simulink model "model1"  (R2023a)
settings: Solver=VariableStepAuto  StartTime=0.0  StopTime=2  RelTol=1e-5
values from neighbouring files (symbols this model uses):
  beta = 0.001    [LR1.m]
  C_m = 1.3    [LR1.m]
  C_w = 3.15    [LR1.m]
  J = 7e-6    (= 7e-06)    [LR1.m]
  L_ov = 0.013    [LR1.m]
  L_ya = 0.0015    [LR1.m]
  R_ya = 8    [LR1.m]
settings Model: Creator=Артём  LastModifiedBy=Артём

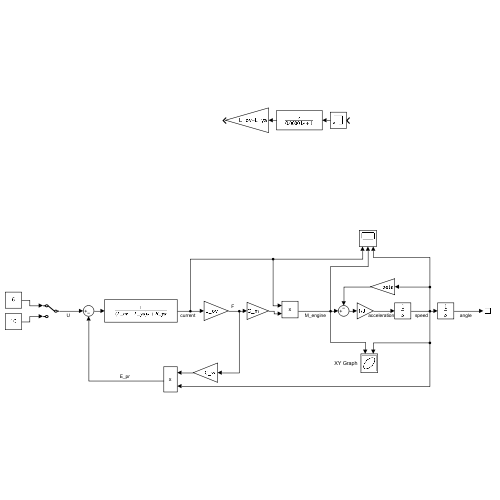
[thumbnail: Simulink's stored preview of the top-level diagram]
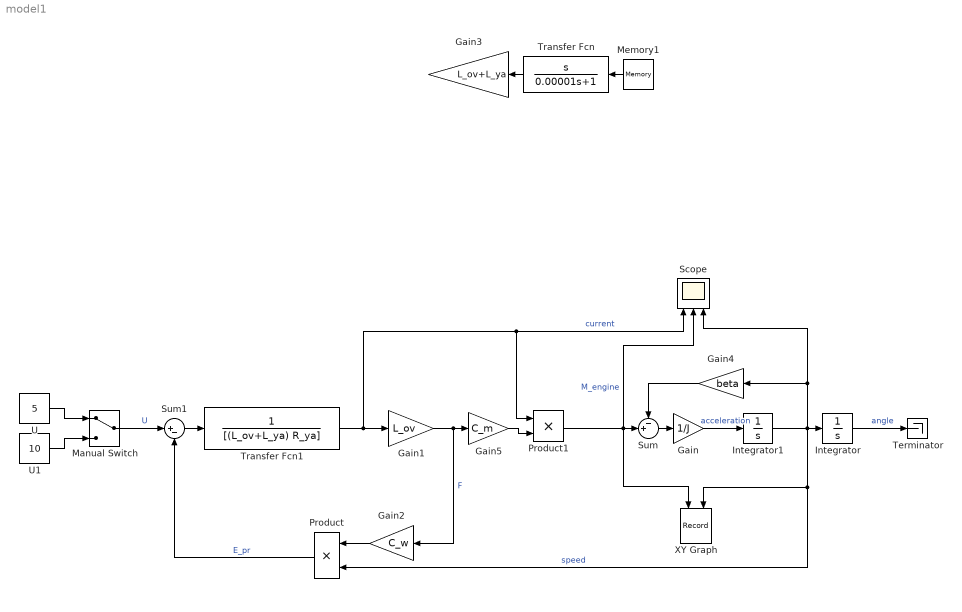
== system model1 ==
  Gain : Gain  Gain=1/J
  Gain1 : Gain  Gain=L_ov
  Gain2 : Gain  Gain=C_w
  Gain3 : Gain  Gain=L_ov+L_ya
  Gain4 : Gain  Gain=beta
  Gain5 : Gain  Gain=C_m
  Integrator : Integrator
  Integrator1 : Integrator  ZeroCross=off
  Manual Switch : ManualSwitch
  Memory1 : Memory
  Product : Product
  Product1 : Product
  Scope : Scope  NumInputPorts=3
  Sum : Sum  Inputs=-+|
  Sum1 : Sum  Inputs=|+-
  Terminator : Terminator
  Transfer Fcn : TransferFcn  Numerator=[1 0]  Denominator=[0.00001 1]
  Transfer Fcn1 : TransferFcn  Denominator=[(L_ov+L_ya) R_ya]
  U : Constant  Value=5
  U1 : Constant  Value=10
  XY Graph : Record  FileSettingsInternal="{\"entries\":[{\"content\":{\"excelSettings\":{\"content\":{},\"type\":\"Streamout.ExcelSettings\"}},\"type\":\"Streamout.FileSettingStorage\",\"uuid\":\"\"}],\"packageUris\":[\"http:\\/\\/schema.mathworks.com\\/mf0\\/streamout_blocks\\/R2020a\"],\"version\":\"1.0\"}"  Layout=[1 1]  SignalsInternal="{\"entries\":[{\"content\":{\"signals\":[{\"content\":{\"blockPath\":[],\"dimensions\":[1],\"domain\":\"\",\"lineColor\":\"#a2142f\",\"plots\":[1],\"port\":1,\"sid\":[\"\"],\"signalID\":431,\"signalName\":\"M_engine\"},\"type\":\"RecordBlkView.Signal\",\"uuid\":\"\"},{\"content\":{\"blockPath\":[],\"dimensions\":[1],\"domain\":\"\",\"lineColor\":\"#139fff\",\"plots\":[1],\"port\":2,\"sid\":[\"\"],\"signalID\":435,\"signalName\":\"speed\"},\"type\":\"RecordBlkView.Signal\",\"uuid\":\"\"}]},\"type\":\"RecordBlkView.InputSignals\",\"uuid\":\"\"}],\"packageUris\":[\"http:\\/\\/schema.mathworks.com\\/mf0\\/streamout_blocks\\/R2020a\"],\"version\":\"1.0\"}"  VisualizationBindings="{\"xyplotplugin\":{\"info\":[{\"series\":[{\"bindingParametersList\":[{\"parameter\":\"X-Axis\",\"signalID\":431,\"signalName\":\"M_engine\"},{\"parameter\":\"Y-Axis\",\"signalID\":435,\"signalName\":\"speed\"}],\"seriesID\":53410}],\"subplotID\":1}]}}"  CompatibilityTag=XY
  wires:
  Integrator/1 -> Terminator/1  "angle"
  U/1 -> Manual Switch/1
  Gain/1 -> Integrator1/1  "acceleration"
  Transfer Fcn/1 -> Gain3/1
  Product/1 -> Sum1/2  "E_pr"
  U1/1 -> Manual Switch/2
  Manual Switch/1 -> Sum1/1  "U"
  Sum1/1 -> Transfer Fcn1/1
  Gain1/1 -> Gain5/1, Gain2/1  "F"
  Gain2/1 -> Product/1
  Memory1/1 -> Transfer Fcn/1
  Transfer Fcn1/1 -> Gain1/1, Product1/1, Scope/1  "current"
  Integrator1/1 -> Gain4/1, Scope/3, XY Graph/2, Product/2, Integrator/1  "speed"
  Gain4/1 -> Sum/1
  Product1/1 -> Sum/2, Scope/2, XY Graph/1  "M_engine"
  Gain5/1 -> Product1/2
  Sum/1 -> Gain/1
